simulink model "Exercise2Matlab"  (R2019a)
settings: Solver=VariableStepAuto  StartTime=0.0  StopTime=10.0  RelTol=1e-3
settings Model: Creator=G5  LastModifiedBy=G5

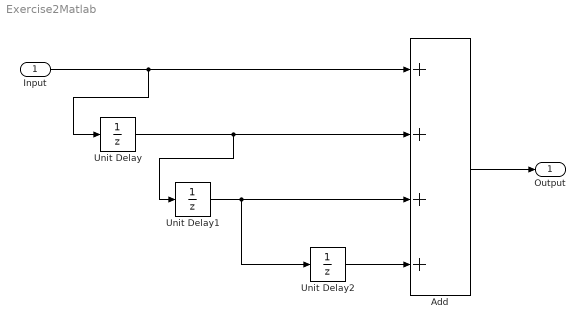
== system Exercise2Matlab ==
  Input : Inport
  Add : Sum  Inputs=++++
  Unit Delay : UnitDelay  SampleTime=-1  HasFrameUpgradeWarning=on
  Unit Delay1 : UnitDelay  SampleTime=-1  HasFrameUpgradeWarning=on
  Unit Delay2 : UnitDelay  SampleTime=-1  HasFrameUpgradeWarning=on
  Output : Outport
  wires:
  Unit Delay/1 -> Unit Delay1/1, Add/2
  Input/1 -> Unit Delay/1, Add/1
  Unit Delay1/1 -> Unit Delay2/1, Add/3
  Unit Delay2/1 -> Add/4
  Add/1 -> Output/1
